simulink model "controller1"  (R2022a)
settings: Solver=VariableStepAuto  StartTime=0.0  StopTime=44  MaxStep=1e-3  MinStep=1e-6  RelTol=1e-3
libraries: dspswit3 x1
(part 2 of 2)

== matlab function controller1/Subsystem/MATLAB Function ==
  data: q input; f_matrix output; qd input; g_matrix output
function [f_matrix,g_matrix] = fcn(q,qd)
% q1=q(1);
q2=q(2);q3=q(3);
dq1=qd(1);dq2=qd(2);dq3=qd(3);

Izz1=0.192;
Ixx3=0.063; Iyy3=0.061; Izz3= 0.02;
Ixx2=0.0027; Iyy2=0.0024; Izz2=0.0004;

g_matrix =[                                                                                                                                                                                                                                                                                                                                                                                                                                                                                                                                                                                                                                                                                                                                                                                                                                                                                                                                                                                                                                                                                             0,                                                                                                                                                                                                             -(- sin(q2)*dq1^2*cos(q2)*sin(q3)^2 + sin(q2)*dq1^2*cos(q2) + dq2*cos(q3)*sin(q2)*dq1*cos(q2)^2*sin(q3) + dq2*sin(q2)*dq1*cos(q2)*sin(q3)^2 - dq2*sin(q2)*dq1*cos(q2))/(Iyy3*Izz1*Izz3 + Izz1*Izz2*Izz3 + Ixx2*Iyy3*Izz3*cos(q2)^2 + Ixx2*Izz2*Izz3*cos(q2)^2 + Ixx3*Izz1*Izz3*sin(q3)^2 + Iyy2*Iyy3*Izz3*sin(q2)^2 + Iyy2*Izz2*Izz3*sin(q2)^2 - Iyy3*Izz1*Izz3*sin(q3)^2 + Iyy3^2*Izz3*cos(q2)^2*sin(q3)^2 - Iyy3^2*Izz3*cos(q2)^2*sin(q3)^4 + Ixx3*Iyy3*Izz3*cos(q2)^2*cos(q3)^2 + Ixx3*Izz2*Izz3*cos(q2)^2*cos(q3)^2 + Ixx2*Ixx3*Izz3*cos(q2)^2*sin(q3)^2 - Ixx2*Iyy3*Izz3*cos(q2)^2*sin(q3)^2 + Ixx3*Iyy3*Izz3*cos(q2)^2*sin(q3)^4 + Iyy3*Izz2*Izz3*cos(q2)^2*sin(q3)^2 + Ixx3*Iyy2*Izz3*sin(q2)^2*sin(q3)^2 - Iyy2*Iyy3*Izz3*sin(q2)^2*sin(q3)^2 - Iyy3^2*Izz3*cos(q2)^2*cos(q3)^2*sin(q3)^2 + Ixx3*Iyy3*Izz3*cos(q2)^2*cos(q3)^2*sin(q3)^2),                                                                    (dq1^2*cos(q2)*sin(q2) - (dq1*dq2*cos(q2))/2 + (dq1*dq3*cos(q2))/2 - dq1^2*cos(q2)*sin(q2)*sin(q3)^2 + (dq1*dq2*cos(q2)*sin(q3)^2)/2 - (dq1*dq3*cos(q2)*sin(q3)^2)/2 - dq1*dq2*cos(q2)*sin(q2) - (dq1*dq3*cos(q2)*sin(q2))/2 + (dq2*dq3*cos(q2)*sin(q2))/2 + (dq1*dq2*cos(q2)^2*cos(q3)*sin(q3))/2 + (dq2*dq3*cos(q2)^2*cos(q3)*sin(q3))/2 + dq1*dq2*cos(q2)*sin(q2)*sin(q3)^2 + (dq1*dq3*cos(q2)*sin(q2)*sin(q3)^2)/2 - (dq2*dq3*cos(q2)*sin(q2)*sin(q3)^2)/2 + dq1*dq2*cos(q2)^2*cos(q3)*sin(q2)*sin(q3))/(Iyy3*Izz1*Izz3 + Izz1*Izz2*Izz3 + Ixx2*Iyy3*Izz3*cos(q2)^2 + Ixx2*Izz2*Izz3*cos(q2)^2 + Ixx3*Izz1*Izz3*sin(q3)^2 + Iyy2*Iyy3*Izz3*sin(q2)^2 + Iyy2*Izz2*Izz3*sin(q2)^2 - Iyy3*Izz1*Izz3*sin(q3)^2 + Iyy3^2*Izz3*cos(q2)^2*sin(q3)^2 - Iyy3^2*Izz3*cos(q2)^2*sin(q3)^4 + Ixx3*Iyy3*Izz3*cos(q2)^2*cos(q3)^2 + Ixx3*Izz2*Izz3*cos(q2)^2*cos(q3)^2 + Ixx2*Ixx3*Izz3*cos(q2)^2*sin(q3)^2 - Ixx2*Iyy3*Izz3*cos(q2)^2*sin(q3)^2 + Ixx3*Iyy3*Izz3*cos(q2)^2*sin(q3)^4 + Iyy3*Izz2*Izz3*cos(q2)^2*sin(q3)^2 + Ixx3*Iyy2*Izz3*sin(q2)^2*sin(q3)^2 - Iyy2*Iyy3*Izz3*sin(q2)^2*sin(q3)^2 - Iyy3^2*Izz3*cos(q2)^2*cos(q3)^2*sin(q3)^2 + Ixx3*Iyy3*Izz3*cos(q2)^2*cos(q3)^2*sin(q3)^2),                                                                                                                                                                                                                                                                                                                                                                                                                                                                                                                                                                                                                                                                                                                                                                                                                                            0,                                                                                                                                                                                                  (dq1*dq2*cos(q2)*sin(q2)*sin(q3)^2 - dq1^2*cos(q2)*sin(q2)*sin(q3)^2 + dq1*dq2*cos(q2)^2*cos(q3)*sin(q2)*sin(q3))/(Iyy3*Izz1*Izz3 + Izz1*Izz2*Izz3 + Ixx2*Iyy3*Izz3*cos(q2)^2 + Ixx2*Izz2*Izz3*cos(q2)^2 + Ixx3*Izz1*Izz3*sin(q3)^2 + Iyy2*Iyy3*Izz3*sin(q2)^2 + Iyy2*Izz2*Izz3*sin(q2)^2 - Iyy3*Izz1*Izz3*sin(q3)^2 + Iyy3^2*Izz3*cos(q2)^2*sin(q3)^2 - Iyy3^2*Izz3*cos(q2)^2*sin(q3)^4 + Ixx3*Iyy3*Izz3*cos(q2)^2*cos(q3)^2 + Ixx3*Izz2*Izz3*cos(q2)^2*cos(q3)^2 + Ixx2*Ixx3*Izz3*cos(q2)^2*sin(q3)^2 - Ixx2*Iyy3*Izz3*cos(q2)^2*sin(q3)^2 + Ixx3*Iyy3*Izz3*cos(q2)^2*sin(q3)^4 + Iyy3*Izz2*Izz3*cos(q2)^2*sin(q3)^2 + Ixx3*Iyy2*Izz3*sin(q2)^2*sin(q3)^2 - Iyy2*Iyy3*Izz3*sin(q2)^2*sin(q3)^2 - Iyy3^2*Izz3*cos(q2)^2*cos(q3)^2*sin(q3)^2 + Ixx3*Iyy3*Izz3*cos(q2)^2*cos(q3)^2*sin(q3)^2),                                                                                                                                                                                                                                                                                                       -(dq1*dq2*cos(q2)*sin(q2)*sin(q3)^2 - dq1^2*cos(q2)*sin(q2)*sin(q3)^2 + dq1*dq2*cos(q2)^2*cos(q3)*sin(q2)*sin(q3))/(Iyy3*Izz1*Izz3 + Izz1*Izz2*Izz3 + Ixx2*Iyy3*Izz3*cos(q2)^2 + Ixx2*Izz2*Izz3*cos(q2)^2 + Ixx3*Izz1*Izz3*sin(q3)^2 + Iyy2*Iyy3*Izz3*sin(q2)^2 + Iyy2*Izz2*Izz3*sin(q2)^2 - Iyy3*Izz1*Izz3*sin(q3)^2 + Iyy3^2*Izz3*cos(q2)^2*sin(q3)^2 - Iyy3^2*Izz3*cos(q2)^2*sin(q3)^4 + Ixx3*Iyy3*Izz3*cos(q2)^2*cos(q3)^2 + Ixx3*Izz2*Izz3*cos(q2)^2*cos(q3)^2 + Ixx2*Ixx3*Izz3*cos(q2)^2*sin(q3)^2 - Ixx2*Iyy3*Izz3*cos(q2)^2*sin(q3)^2 + Ixx3*Iyy3*Izz3*cos(q2)^2*sin(q3)^4 + Iyy3*Izz2*Izz3*cos(q2)^2*sin(q3)^2 + Ixx3*Iyy2*Izz3*sin(q2)^2*sin(q3)^2 - Iyy2*Iyy3*Izz3*sin(q2)^2*sin(q3)^2 - Iyy3^2*Izz3*cos(q2)^2*cos(q3)^2*sin(q3)^2 + Ixx3*Iyy3*Izz3*cos(q2)^2*cos(q3)^2*sin(q3)^2),                                                                      (cos(q2)*sin(q2)*dq1^2 - dq2*cos(q2)*sin(q2)*dq1)/(Iyy3*Izz1*Izz3 + Izz1*Izz2*Izz3 + Ixx2*Iyy3*Izz3*cos(q2)^2 + Ixx2*Izz2*Izz3*cos(q2)^2 + Ixx3*Izz1*Izz3*sin(q3)^2 + Iyy2*Iyy3*Izz3*sin(q2)^2 + Iyy2*Izz2*Izz3*sin(q2)^2 - Iyy3*Izz1*Izz3*sin(q3)^2 + Iyy3^2*Izz3*cos(q2)^2*sin(q3)^2 - Iyy3^2*Izz3*cos(q2)^2*sin(q3)^4 + Ixx3*Iyy3*Izz3*cos(q2)^2*cos(q3)^2 + Ixx3*Izz2*Izz3*cos(q2)^2*cos(q3)^2 + Ixx2*Ixx3*Izz3*cos(q2)^2*sin(q3)^2 - Ixx2*Iyy3*Izz3*cos(q2)^2*sin(q3)^2 + Ixx3*Iyy3*Izz3*cos(q2)^2*sin(q3)^4 + Iyy3*Izz2*Izz3*cos(q2)^2*sin(q3)^2 + Ixx3*Iyy2*Izz3*sin(q2)^2*sin(q3)^2 - Iyy2*Iyy3*Izz3*sin(q2)^2*sin(q3)^2 - Iyy3^2*Izz3*cos(q2)^2*cos(q3)^2*sin(q3)^2 + Ixx3*Iyy3*Izz3*cos(q2)^2*cos(q3)^2*sin(q3)^2)
                                                                                                                                                                                                                                                                                                                                                                                                                                                                                                                                                                                                                                                                                                                                                                                                                                                                                                                                                                                                                                                                                             0, -((dq2*dq3*cos(q2)^3)/2 - (dq1*dq2*cos(q2)^3)/2 + dq2^2*cos(q2)^2*cos(q3)*sin(q3) + dq1*dq2*cos(q2)^3*sin(q2) + dq1*dq2*cos(q2)^3*cos(q3)^2 - dq2*dq3*cos(q2)^3*cos(q3)^2 - dq2*dq3*cos(q2)^2*cos(q3)*sin(q3) - dq1*dq2*cos(q2)^3*cos(q3)^2*sin(q2) + dq1*dq2*cos(q2)^3*sin(q2)*sin(q3)^2 + dq1^2*cos(q2)^2*cos(q3)*sin(q2)*sin(q3) - 2*dq1*dq2*cos(q2)^2*cos(q3)*sin(q2)*sin(q3))/(Iyy3*Izz1*Izz3 + Izz1*Izz2*Izz3 + Ixx2*Iyy3*Izz3*cos(q2)^2 + Ixx2*Izz2*Izz3*cos(q2)^2 + Ixx3*Izz1*Izz3*sin(q3)^2 + Iyy2*Iyy3*Izz3*sin(q2)^2 + Iyy2*Izz2*Izz3*sin(q2)^2 - Iyy3*Izz1*Izz3*sin(q3)^2 + Iyy3^2*Izz3*cos(q2)^2*sin(q3)^2 - Iyy3^2*Izz3*cos(q2)^2*sin(q3)^4 + Ixx3*Iyy3*Izz3*cos(q2)^2*cos(q3)^2 + Ixx3*Izz2*Izz3*cos(q2)^2*cos(q3)^2 + Ixx2*Ixx3*Izz3*cos(q2)^2*sin(q3)^2 - Ixx2*Iyy3*Izz3*cos(q2)^2*sin(q3)^2 + Ixx3*Iyy3*Izz3*cos(q2)^2*sin(q3)^4 + Iyy3*Izz2*Izz3*cos(q2)^2*sin(q3)^2 + Ixx3*Iyy2*Izz3*sin(q2)^2*sin(q3)^2 - Iyy2*Iyy3*Izz3*sin(q2)^2*sin(q3)^2 - Iyy3^2*Izz3*cos(q2)^2*cos(q3)^2*sin(q3)^2 + Ixx3*Iyy3*Izz3*cos(q2)^2*cos(q3)^2*sin(q3)^2),                                                                                                                                                                                                ((dq1*dq2*cos(q2)^3*sin(q3)^2)/2 + (dq2*dq3*cos(q2)^3*sin(q3)^2)/2 - (dq1*dq2*cos(q2)^2*cos(q3)*sin(q3))/2 + (dq1*dq3*cos(q2)^2*cos(q3)*sin(q3))/2 + dq1*dq2*cos(q2)^3*sin(q2)*sin(q3)^2 + dq1^2*cos(q2)^2*cos(q3)*sin(q2)*sin(q3) - dq1*dq2*cos(q2)^2*cos(q3)*sin(q2)*sin(q3) - (dq1*dq3*cos(q2)^2*cos(q3)*sin(q2)*sin(q3))/2 + (dq2*dq3*cos(q2)^2*cos(q3)*sin(q2)*sin(q3))/2)/(Iyy3*Izz1*Izz3 + Izz1*Izz2*Izz3 + Ixx2*Iyy3*Izz3*cos(q2)^2 + Ixx2*Izz2*Izz3*cos(q2)^2 + Ixx3*Izz1*Izz3*sin(q3)^2 + Iyy2*Iyy3*Izz3*sin(q2)^2 + Iyy2*Izz2*Izz3*sin(q2)^2 - Iyy3*Izz1*Izz3*sin(q3)^2 + Iyy3^2*Izz3*cos(q2)^2*sin(q3)^2 - Iyy3^2*Izz3*cos(q2)^2*sin(q3)^4 + Ixx3*Iyy3*Izz3*cos(q2)^2*cos(q3)^2 + Ixx3*Izz2*Izz3*cos(q2)^2*cos(q3)^2 + Ixx2*Ixx3*Izz3*cos(q2)^2*sin(q3)^2 - Ixx2*Iyy3*Izz3*cos(q2)^2*sin(q3)^2 + Ixx3*Iyy3*Izz3*cos(q2)^2*sin(q3)^4 + Iyy3*Izz2*Izz3*cos(q2)^2*sin(q3)^2 + Ixx3*Iyy2*Izz3*sin(q2)^2*sin(q3)^2 - Iyy2*Iyy3*Izz3*sin(q2)^2*sin(q3)^2 - Iyy3^2*Izz3*cos(q2)^2*cos(q3)^2*sin(q3)^2 + Ixx3*Iyy3*Izz3*cos(q2)^2*cos(q3)^2*sin(q3)^2),                                                                                                                                                                                                                                                                                                                                                                                                                                                                                                                                                                                                                                                                                                                                                                                                                                            0, -((dq1*dq2*cos(q2)^3)/2 - (dq2*dq3*cos(q2)^3)/2 - dq2^2*cos(q2)^2*cos(q3)*sin(q3) - dq1*dq2*cos(q2)^3*cos(q3)^2 + dq2*dq3*cos(q2)^3*cos(q3)^2 + dq2*dq3*cos(q2)^2*cos(q3)*sin(q3) + 2*dq1*dq2*cos(q2)^3*cos(q3)^2*sin(q2) - dq1^2*cos(q2)^2*cos(q3)*sin(q2)*sin(q3) + 2*dq1*dq2*cos(q2)^2*cos(q3)*sin(q2)*sin(q3))/(Iyy3*Izz1*Izz3 + Izz1*Izz2*Izz3 + Ixx2*Iyy3*Izz3*cos(q2)^2 + Ixx2*Izz2*Izz3*cos(q2)^2 + Ixx3*Izz1*Izz3*sin(q3)^2 + Iyy2*Iyy3*Izz3*sin(q2)^2 + Iyy2*Izz2*Izz3*sin(q2)^2 - Iyy3*Izz1*Izz3*sin(q3)^2 + Iyy3^2*Izz3*cos(q2)^2*sin(q3)^2 - Iyy3^2*Izz3*cos(q2)^2*sin(q3)^4 + Ixx3*Iyy3*Izz3*cos(q2)^2*cos(q3)^2 + Ixx3*Izz2*Izz3*cos(q2)^2*cos(q3)^2 + Ixx2*Ixx3*Izz3*cos(q2)^2*sin(q3)^2 - Ixx2*Iyy3*Izz3*cos(q2)^2*sin(q3)^2 + Ixx3*Iyy3*Izz3*cos(q2)^2*sin(q3)^4 + Iyy3*Izz2*Izz3*cos(q2)^2*sin(q3)^2 + Ixx3*Iyy2*Izz3*sin(q2)^2*sin(q3)^2 - Iyy2*Iyy3*Izz3*sin(q2)^2*sin(q3)^2 - Iyy3^2*Izz3*cos(q2)^2*cos(q3)^2*sin(q3)^2 + Ixx3*Iyy3*Izz3*cos(q2)^2*cos(q3)^2*sin(q3)^2), -((dq1*dq2*cos(q2)*sin(q2)^2)/2 - dq2^2*cos(q3)*sin(q2)^2*sin(q3) - (dq2*dq3*cos(q2)*sin(q2)^2)/2 + dq1*dq2*cos(q3)*sin(q2)^3*sin(q3) + dq2*dq3*cos(q3)*sin(q2)^2*sin(q3) - dq1*dq2*cos(q2)*cos(q3)^2*sin(q2)^2 + dq1*dq2*cos(q2)*cos(q3)^2*sin(q2)^3 - dq1*dq2*cos(q2)^3*cos(q3)^2*sin(q2) + dq2*dq3*cos(q2)*cos(q3)^2*sin(q2)^2 + dq1^2*cos(q2)^2*cos(q3)*sin(q2)*sin(q3) - dq1*dq2*cos(q2)^2*cos(q3)*sin(q2)*sin(q3))/(Iyy3*Izz1*Izz3 + Izz1*Izz2*Izz3 + Ixx2*Iyy3*Izz3*cos(q2)^2 + Ixx2*Izz2*Izz3*cos(q2)^2 + Ixx3*Izz1*Izz3*sin(q3)^2 + Iyy2*Iyy3*Izz3*sin(q2)^2 + Iyy2*Izz2*Izz3*sin(q2)^2 - Iyy3*Izz1*Izz3*sin(q3)^2 + Iyy3^2*Izz3*cos(q2)^2*sin(q3)^2 - Iyy3^2*Izz3*cos(q2)^2*sin(q3)^4 + Ixx3*Iyy3*Izz3*cos(q2)^2*cos(q3)^2 + Ixx3*Izz2*Izz3*cos(q2)^2*cos(q3)^2 + Ixx2*Ixx3*Izz3*cos(q2)^2*sin(q3)^2 - Ixx2*Iyy3*Izz3*cos(q2)^2*sin(q3)^2 + Ixx3*Iyy3*Izz3*cos(q2)^2*sin(q3)^4 + Iyy3*Izz2*Izz3*cos(q2)^2*sin(q3)^2 + Ixx3*Iyy2*Izz3*sin(q2)^2*sin(q3)^2 - Iyy2*Iyy3*Izz3*sin(q2)^2*sin(q3)^2 - Iyy3^2*Izz3*cos(q2)^2*cos(q3)^2*sin(q3)^2 + Ixx3*Iyy3*Izz3*cos(q2)^2*cos(q3)^2*sin(q3)^2),                                                                                                                                                                                                                                                                                                                                                                                                                                                                                                                                                                                                                                                                                                                                                                                                 0
((dq1*dq3*cos(q2)^3)/2 + (dq2*dq3*cos(q2)^3)/2 - dq1*dq3*cos(q2)^3*cos(q3)^2 - dq2*dq3*cos(q2)^3*cos(q3)^2 - (dq1*dq3*cos(q2)^3*sin(q3)^2)/2 - (dq2*dq3*cos(q2)^3*sin(q3)^2)/2 - dq2*dq3*cos(q2)^2*cos(q3)*sin(q3) + dq1*dq3*cos(q2)^4*cos(q3)*sin(q3) + dq2*dq3*cos(q2)^2*cos(q3)*sin(q3)^3 - dq1*dq3*cos(q2)^4*cos(q3)*sin(q3)^3 + dq1*dq3*cos(q2)^3*cos(q3)^2*sin(q3)^2 + dq2*dq3*cos(q2)^3*cos(q3)^2*sin(q3)^2)/(Iyy3*Izz1*Izz3 + Izz1*Izz2*Izz3 + Ixx2*Iyy3*Izz3*cos(q2)^2 + Ixx2*Izz2*Izz3*cos(q2)^2 + Ixx3*Izz1*Izz3*sin(q3)^2 + Iyy2*Iyy3*Izz3*sin(q2)^2 + Iyy2*Izz2*Izz3*sin(q2)^2 - Iyy3*Izz1*Izz3*sin(q3)^2 + Iyy3^2*Izz3*cos(q2)^2*sin(q3)^2 - Iyy3^2*Izz3*cos(q2)^2*sin(q3)^4 + Ixx3*Iyy3*Izz3*cos(q2)^2*cos(q3)^2 + Ixx3*Izz2*Izz3*cos(q2)^2*cos(q3)^2 + Ixx2*Ixx3*Izz3*cos(q2)^2*sin(q3)^2 - Ixx2*Iyy3*Izz3*cos(q2)^2*sin(q3)^2 + Ixx3*Iyy3*Izz3*cos(q2)^2*sin(q3)^4 + Iyy3*Izz2*Izz3*cos(q2)^2*sin(q3)^2 + Ixx3*Iyy2*Izz3*sin(q2)^2*sin(q3)^2 - Iyy2*Iyy3*Izz3*sin(q2)^2*sin(q3)^2 - Iyy3^2*Izz3*cos(q2)^2*cos(q3)^2*sin(q3)^2 + Ixx3*Iyy3*Izz3*cos(q2)^2*cos(q3)^2*sin(q3)^2),                                                                                  (dq1^2*cos(q2)*sin(q2)^2 + (dq1*dq3*cos(q2)^3)/2 - (dq2*dq3*cos(q2)^3)/2 - dq1*dq2*cos(q2)*sin(q2)^2 - dq1^2*cos(q2)*sin(q2)^2*sin(q3)^2 - (dq1*dq3*cos(q2)^3*sin(q3)^2)/2 + (dq2*dq3*cos(q2)^3*sin(q3)^2)/2 + dq1*dq2*cos(q2)*sin(q2)^2*sin(q3)^2 + dq1*dq2*cos(q2)^2*cos(q3)*sin(q2)^2*sin(q3))/(Iyy3*Izz1*Izz3 + Izz1*Izz2*Izz3 + Ixx2*Iyy3*Izz3*cos(q2)^2 + Ixx2*Izz2*Izz3*cos(q2)^2 + Ixx3*Izz1*Izz3*sin(q3)^2 + Iyy2*Iyy3*Izz3*sin(q2)^2 + Iyy2*Izz2*Izz3*sin(q2)^2 - Iyy3*Izz1*Izz3*sin(q3)^2 + Iyy3^2*Izz3*cos(q2)^2*sin(q3)^2 - Iyy3^2*Izz3*cos(q2)^2*sin(q3)^4 + Ixx3*Iyy3*Izz3*cos(q2)^2*cos(q3)^2 + Ixx3*Izz2*Izz3*cos(q2)^2*cos(q3)^2 + Ixx2*Ixx3*Izz3*cos(q2)^2*sin(q3)^2 - Ixx2*Iyy3*Izz3*cos(q2)^2*sin(q3)^2 + Ixx3*Iyy3*Izz3*cos(q2)^2*sin(q3)^4 + Iyy3*Izz2*Izz3*cos(q2)^2*sin(q3)^2 + Ixx3*Iyy2*Izz3*sin(q2)^2*sin(q3)^2 - Iyy2*Iyy3*Izz3*sin(q2)^2*sin(q3)^2 - Iyy3^2*Izz3*cos(q2)^2*cos(q3)^2*sin(q3)^2 + Ixx3*Iyy3*Izz3*cos(q2)^2*cos(q3)^2*sin(q3)^2), -(dq1^2*cos(q2)*sin(q2)^2 - dq1*dq2*cos(q2)*sin(q2)^2 - (dq1*dq3*cos(q2)*sin(q2)^2)/2 + (dq2*dq3*cos(q2)*sin(q2)^2)/2 - dq1^2*cos(q2)*sin(q2)^2*sin(q3)^2 - (dq1*dq2*cos(q2)*sin(q2))/2 + (dq1*dq3*cos(q2)*sin(q2))/2 + (dq1*dq2*cos(q2)*sin(q2)*sin(q3)^2)/2 - (dq1*dq3*cos(q2)*sin(q2)*sin(q3)^2)/2 + dq1*dq2*cos(q2)*sin(q2)^2*sin(q3)^2 + (dq1*dq3*cos(q2)*sin(q2)^2*sin(q3)^2)/2 - (dq2*dq3*cos(q2)*sin(q2)^2*sin(q3)^2)/2 + dq1*dq2*cos(q2)^2*cos(q3)*sin(q2)^2*sin(q3) + (dq1*dq2*cos(q2)^2*cos(q3)*sin(q2)*sin(q3))/2 + (dq2*dq3*cos(q2)^2*cos(q3)*sin(q2)*sin(q3))/2)/(Iyy3*Izz1*Izz3 + Izz1*Izz2*Izz3 + Ixx2*Iyy3*Izz3*cos(q2)^2 + Ixx2*Izz2*Izz3*cos(q2)^2 + Ixx3*Izz1*Izz3*sin(q3)^2 + Iyy2*Iyy3*Izz3*sin(q2)^2 + Iyy2*Izz2*Izz3*sin(q2)^2 - Iyy3*Izz1*Izz3*sin(q3)^2 + Iyy3^2*Izz3*cos(q2)^2*sin(q3)^2 - Iyy3^2*Izz3*cos(q2)^2*sin(q3)^4 + Ixx3*Iyy3*Izz3*cos(q2)^2*cos(q3)^2 + Ixx3*Izz2*Izz3*cos(q2)^2*cos(q3)^2 + Ixx2*Ixx3*Izz3*cos(q2)^2*sin(q3)^2 - Ixx2*Iyy3*Izz3*cos(q2)^2*sin(q3)^2 + Ixx3*Iyy3*Izz3*cos(q2)^2*sin(q3)^4 + Iyy3*Izz2*Izz3*cos(q2)^2*sin(q3)^2 + Ixx3*Iyy2*Izz3*sin(q2)^2*sin(q3)^2 - Iyy2*Iyy3*Izz3*sin(q2)^2*sin(q3)^2 - Iyy3^2*Izz3*cos(q2)^2*cos(q3)^2*sin(q3)^2 + Ixx3*Iyy3*Izz3*cos(q2)^2*cos(q3)^2*sin(q3)^2), ((dq1*dq3*cos(q2))/2 + (dq2*dq3*cos(q2))/2 - dq1*dq3*cos(q2)*cos(q3)^2 - dq2*dq3*cos(q2)*cos(q3)^2 - dq2*dq3*cos(q3)*sin(q3) + dq1*dq3*cos(q2)^2*cos(q3)*sin(q3))/(Iyy3*Izz1*Izz3 + Izz1*Izz2*Izz3 + Ixx2*Iyy3*Izz3*cos(q2)^2 + Ixx2*Izz2*Izz3*cos(q2)^2 + Ixx3*Izz1*Izz3*sin(q3)^2 + Iyy2*Iyy3*Izz3*sin(q2)^2 + Iyy2*Izz2*Izz3*sin(q2)^2 - Iyy3*Izz1*Izz3*sin(q3)^2 + Iyy3^2*Izz3*cos(q2)^2*sin(q3)^2 - Iyy3^2*Izz3*cos(q2)^2*sin(q3)^4 + Ixx3*Iyy3*Izz3*cos(q2)^2*cos(q3)^2 + Ixx3*Izz2*Izz3*cos(q2)^2*cos(q3)^2 + Ixx2*Ixx3*Izz3*cos(q2)^2*sin(q3)^2 - Ixx2*Iyy3*Izz3*cos(q2)^2*sin(q3)^2 + Ixx3*Iyy3*Izz3*cos(q2)^2*sin(q3)^4 + Iyy3*Izz2*Izz3*cos(q2)^2*sin(q3)^2 + Ixx3*Iyy2*Izz3*sin(q2)^2*sin(q3)^2 - Iyy2*Iyy3*Izz3*sin(q2)^2*sin(q3)^2 - Iyy3^2*Izz3*cos(q2)^2*cos(q3)^2*sin(q3)^2 + Ixx3*Iyy3*Izz3*cos(q2)^2*cos(q3)^2*sin(q3)^2),                                                                                                                       -((dq2*dq3*cos(q2)^3*sin(q3)^2)/2 - (dq1*dq3*cos(q2)^3*sin(q3)^2)/2 - dq1^2*cos(q2)*sin(q2)^2*sin(q3)^2 + dq1*dq2*cos(q2)*sin(q2)^2*sin(q3)^2 + dq1*dq2*cos(q2)^2*cos(q3)*sin(q2)^2*sin(q3))/(Iyy3*Izz1*Izz3 + Izz1*Izz2*Izz3 + Ixx2*Iyy3*Izz3*cos(q2)^2 + Ixx2*Izz2*Izz3*cos(q2)^2 + Ixx3*Izz1*Izz3*sin(q3)^2 + Iyy2*Iyy3*Izz3*sin(q2)^2 + Iyy2*Izz2*Izz3*sin(q2)^2 - Iyy3*Izz1*Izz3*sin(q3)^2 + Iyy3^2*Izz3*cos(q2)^2*sin(q3)^2 - Iyy3^2*Izz3*cos(q2)^2*sin(q3)^4 + Ixx3*Iyy3*Izz3*cos(q2)^2*cos(q3)^2 + Ixx3*Izz2*Izz3*cos(q2)^2*cos(q3)^2 + Ixx2*Ixx3*Izz3*cos(q2)^2*sin(q3)^2 - Ixx2*Iyy3*Izz3*cos(q2)^2*sin(q3)^2 + Ixx3*Iyy3*Izz3*cos(q2)^2*sin(q3)^4 + Iyy3*Izz2*Izz3*cos(q2)^2*sin(q3)^2 + Ixx3*Iyy2*Izz3*sin(q2)^2*sin(q3)^2 - Iyy2*Iyy3*Izz3*sin(q2)^2*sin(q3)^2 - Iyy3^2*Izz3*cos(q2)^2*cos(q3)^2*sin(q3)^2 + Ixx3*Iyy3*Izz3*cos(q2)^2*cos(q3)^2*sin(q3)^2),                                                                                                                                                                                                              (dq1*dq2*cos(q2)*sin(q2)^2*sin(q3)^2 - dq1^2*cos(q2)*sin(q2)^2*sin(q3)^2 + (dq1*dq3*cos(q2)*sin(q2)^2*sin(q3)^2)/2 - (dq2*dq3*cos(q2)*sin(q2)^2*sin(q3)^2)/2 + dq1*dq2*cos(q2)^2*cos(q3)*sin(q2)^2*sin(q3))/(Iyy3*Izz1*Izz3 + Izz1*Izz2*Izz3 + Ixx2*Iyy3*Izz3*cos(q2)^2 + Ixx2*Izz2*Izz3*cos(q2)^2 + Ixx3*Izz1*Izz3*sin(q3)^2 + Iyy2*Iyy3*Izz3*sin(q2)^2 + Iyy2*Izz2*Izz3*sin(q2)^2 - Iyy3*Izz1*Izz3*sin(q3)^2 + Iyy3^2*Izz3*cos(q2)^2*sin(q3)^2 - Iyy3^2*Izz3*cos(q2)^2*sin(q3)^4 + Ixx3*Iyy3*Izz3*cos(q2)^2*cos(q3)^2 + Ixx3*Izz2*Izz3*cos(q2)^2*cos(q3)^2 + Ixx2*Ixx3*Izz3*cos(q2)^2*sin(q3)^2 - Ixx2*Iyy3*Izz3*cos(q2)^2*sin(q3)^2 + Ixx3*Iyy3*Izz3*cos(q2)^2*sin(q3)^4 + Iyy3*Izz2*Izz3*cos(q2)^2*sin(q3)^2 + Ixx3*Iyy2*Izz3*sin(q2)^2*sin(q3)^2 - Iyy2*Iyy3*Izz3*sin(q2)^2*sin(q3)^2 - Iyy3^2*Izz3*cos(q2)^2*cos(q3)^2*sin(q3)^2 + Ixx3*Iyy3*Izz3*cos(q2)^2*cos(q3)^2*sin(q3)^2), -(dq1^2*cos(q2)*sin(q2)^2 - dq1*dq2*cos(q2)*sin(q2)^2 - (dq1*dq3*cos(q2)*sin(q2)^2)/2 + (dq2*dq3*cos(q2)*sin(q2)^2)/2)/(Iyy3*Izz1*Izz3 + Izz1*Izz2*Izz3 + Ixx2*Iyy3*Izz3*cos(q2)^2 + Ixx2*Izz2*Izz3*cos(q2)^2 + Ixx3*Izz1*Izz3*sin(q3)^2 + Iyy2*Iyy3*Izz3*sin(q2)^2 + Iyy2*Izz2*Izz3*sin(q2)^2 - Iyy3*Izz1*Izz3*sin(q3)^2 + Iyy3^2*Izz3*cos(q2)^2*sin(q3)^2 - Iyy3^2*Izz3*cos(q2)^2*sin(q3)^4 + Ixx3*Iyy3*Izz3*cos(q2)^2*cos(q3)^2 + Ixx3*Izz2*Izz3*cos(q2)^2*cos(q3)^2 + Ixx2*Ixx3*Izz3*cos(q2)^2*sin(q3)^2 - Ixx2*Iyy3*Izz3*cos(q2)^2*sin(q3)^2 + Ixx3*Iyy3*Izz3*cos(q2)^2*sin(q3)^4 + Iyy3*Izz2*Izz3*cos(q2)^2*sin(q3)^2 + Ixx3*Iyy2*Izz3*sin(q2)^2*sin(q3)^2 - Iyy2*Iyy3*Izz3*sin(q2)^2*sin(q3)^2 - Iyy3^2*Izz3*cos(q2)^2*cos(q3)^2*sin(q3)^2 + Ixx3*Iyy3*Izz3*cos(q2)^2*cos(q3)^2*sin(q3)^2)];
 

f_matrix =[
                                                                                                                                                                                                                                                                                                                                                                                                                                                                                                                                                                                                                                                                                                                                                                                                                                                                                                                                                                                                                                                                                                                                                                                                                                                                                                                                                                                                                                                                                                                                                                                                                                                                                                                                                                                                                                                                                                                                                                                                                                                                                                                                                                                                                                                                                                                                                      -(dq1*((Izz3*dq1*(Iyy3 + Izz2 + Ixx3*sin(q3)^2 - Iyy3*sin(q3)^2)*(Ixx3*sin(2*q2 + 2*q3) - Iyy3*sin(2*q2 + 2*q3) + 2*Ixx2*sin(2*q2) + Ixx3*sin(2*q2) + Ixx3*sin(2*q3) - 2*Iyy2*sin(2*q2) + Iyy3*sin(2*q2) - Iyy3*sin(2*q3) - 2*Izz3*sin(2*q2)))/4 + (Izz3*dq3*cos(q2)*sin(q2)*(Iyy3 + Izz2 + Ixx3*sin(q3)^2 - Iyy3*sin(q3)^2)*(Iyy3 - Ixx3 + Izz3 + 2*Ixx3*cos(q3)^2 - 2*Iyy3*cos(q3)^2 - 2*Ixx3*cos(q2)*cos(q3)*sin(q3) + 2*Iyy3*cos(q2)*cos(q3)*sin(q3)))/2 + (Izz3*dq2*cos(q2)*cos(q3)*sin(q3)*(Ixx3 - Iyy3)*(2*Izz3*cos(q2) - 2*Ixx2*sin(2*q2) - Ixx3*sin(2*q2) + 2*Iyy2*sin(2*q2) - Iyy3*sin(2*q2) + 2*Izz3*sin(2*q2) - Ixx3*cos(2*q3)*sin(2*q2) + Iyy3*cos(2*q3)*sin(2*q2) + 2*Ixx3*cos(2*q3)*cos(q2) - 2*Iyy3*cos(2*q3)*cos(q2) - 2*Ixx3*sin(2*q3)*sin(q2) + 2*Iyy3*sin(2*q3)*sin(q2)))/4) + dq2*((Izz3*dq1*cos(q2)*(Iyy3 + Izz2 + Ixx3*sin(q3)^2 - Iyy3*sin(q3)^2)*(Ixx3 - Iyy3 + Izz3 - 2*Ixx2*sin(q2) + 2*Iyy2*sin(q2) - 2*Iyy3*sin(q2) + 2*Izz3*sin(q2) - 2*Ixx3*cos(q3)^2 + 2*Iyy3*cos(q3)^2 - 2*Ixx3*cos(q3)^2*sin(q2) + 2*Iyy3*cos(q3)^2*sin(q2)))/2 - (Izz3*dq3*sin(q2)*(Iyy3 + Izz2 + Ixx3*sin(q3)^2 - Iyy3*sin(q3)^2)*(Ixx3*cos(q2) - Iyy3*cos(q2) + Izz3*cos(q2) - Ixx3*sin(2*q3) + Iyy3*sin(2*q3) - 2*Ixx3*cos(q2)*cos(q3)^2 + 2*Iyy3*cos(q2)*cos(q3)^2))/2 + (Izz3*dq2*sin(2*q3)*cos(q2)*cos(q3)*sin(q3)*(Ixx3 - Iyy3)^2)/2) - dq3*((Izz3*dq1*cos(q2)*(Iyy3 + Izz2 + Ixx3*sin(q3)^2 - Iyy3*sin(q3)^2)*(Ixx3 - Iyy3 + Izz3 - 2*Ixx3*cos(q3)^2 + 2*Iyy3*cos(q3)^2 + 2*Ixx3*cos(q2)*cos(q3)*sin(q3) - 2*Iyy3*cos(q2)*cos(q3)*sin(q3)))/2 - (Izz3*dq2*cos(q2)*cos(q3)*sin(q3)*(Ixx3 - Iyy3)*(Ixx3*cos(q2) - Iyy3*cos(q2) + Izz3*cos(q2) - Ixx3*sin(2*q3) + Iyy3*sin(2*q3) - 2*Ixx3*cos(q2)*cos(q3)^2 + 2*Iyy3*cos(q2)*cos(q3)^2))/2) + Iyy3*Izz3^2*(dq1^2*cos(q2)*sin(q2) - (dq1*dq2*cos(q2))/2 + (dq1*dq3*cos(q2))/2 - dq1^2*cos(q2)*sin(q2)*sin(q3)^2 + (dq1*dq2*cos(q2)*sin(q3)^2)/2 - (dq1*dq3*cos(q2)*sin(q3)^2)/2 - dq1*dq2*cos(q2)*sin(q2) - (dq1*dq3*cos(q2)*sin(q2))/2 + (dq2*dq3*cos(q2)*sin(q2))/2 + (dq1*dq2*cos(q2)^2*cos(q3)*sin(q3))/2 + (dq2*dq3*cos(q2)^2*cos(q3)*sin(q3))/2 + dq1*dq2*cos(q2)*sin(q2)*sin(q3)^2 + (dq1*dq3*cos(q2)*sin(q2)*sin(q3)^2)/2 - (dq2*dq3*cos(q2)*sin(q2)*sin(q3)^2)/2 + dq1*dq2*cos(q2)^2*cos(q3)*sin(q2)*sin(q3)) + Iyy2*Izz2*Izz3*(cos(q2)*sin(q2)*dq1^2 - dq2*cos(q2)*sin(q2)*dq1) - Ixx2*Iyy3*Izz3*(- sin(q2)*dq1^2*cos(q2)*sin(q3)^2 + sin(q2)*dq1^2*cos(q2) + dq2*cos(q3)*sin(q2)*dq1*cos(q2)^2*sin(q3) + dq2*sin(q2)*dq1*cos(q2)*sin(q3)^2 - dq2*sin(q2)*dq1*cos(q2)) + Ixx2*Ixx3*Izz3*(dq1*dq2*cos(q2)*sin(q2)*sin(q3)^2 - dq1^2*cos(q2)*sin(q2)*sin(q3)^2 + dq1*dq2*cos(q2)^2*cos(q3)*sin(q2)*sin(q3)) - Ixx3*Iyy2*Izz3*(dq1*dq2*cos(q2)*sin(q2)*sin(q3)^2 - dq1^2*cos(q2)*sin(q2)*sin(q3)^2 + dq1*dq2*cos(q2)^2*cos(q3)*sin(q2)*sin(q3)))/(Iyy3*Izz1*Izz3 + Izz1*Izz2*Izz3 + Ixx2*Iyy3*Izz3*cos(q2)^2 + Ixx2*Izz2*Izz3*cos(q2)^2 + Ixx3*Izz1*Izz3*sin(q3)^2 + Iyy2*Iyy3*Izz3*sin(q2)^2 + Iyy2*Izz2*Izz3*sin(q2)^2 - Iyy3*Izz1*Izz3*sin(q3)^2 + Iyy3^2*Izz3*cos(q2)^2*sin(q3)^2 - Iyy3^2*Izz3*cos(q2)^2*sin(q3)^4 + Ixx3*Iyy3*Izz3*cos(q2)^2*cos(q3)^2 + Ixx3*Izz2*Izz3*cos(q2)^2*cos(q3)^2 + Ixx2*Ixx3*Izz3*cos(q2)^2*sin(q3)^2 - Ixx2*Iyy3*Izz3*cos(q2)^2*sin(q3)^2 + Ixx3*Iyy3*Izz3*cos(q2)^2*sin(q3)^4 + Iyy3*Izz2*Izz3*cos(q2)^2*sin(q3)^2 + Ixx3*Iyy2*Izz3*sin(q2)^2*sin(q3)^2 - Iyy2*Iyy3*Izz3*sin(q2)^2*sin(q3)^2 - Iyy3^2*Izz3*cos(q2)^2*cos(q3)^2*sin(q3)^2 + Ixx3*Iyy3*Izz3*cos(q2)^2*cos(q3)^2*sin(q3)^2)
                                                                                                                                                                                                                                                                                                                                                                                                                                                                                                                                                                                                                                                                                                                                                                                                                                                                                                                                                                                                                                                                                                                                                                                                                                                                                                                                                                                                                                                                                                                                                                                                                                                     (dq1*((dq2*(Ixx3*Izz3*cos(q2)^2*cos(q3)^2 + Iyy3*Izz3*cos(q2)^2*sin(q3)^2 + Ixx2*Izz3*cos(q2)^2 + Iyy2*Izz3*sin(q2)^2 + Izz1*Izz3)*(2*Izz3*cos(q2) - 2*Ixx2*sin(2*q2) - Ixx3*sin(2*q2) + 2*Iyy2*sin(2*q2) - Iyy3*sin(2*q2) + 2*Izz3*sin(2*q2) - Ixx3*cos(2*q3)*sin(2*q2) + Iyy3*cos(2*q3)*sin(2*q2) + 2*Ixx3*cos(2*q3)*cos(q2) - 2*Iyy3*cos(2*q3)*cos(q2) - 2*Ixx3*sin(2*q3)*sin(q2) + 2*Iyy3*sin(2*q3)*sin(q2)))/4 + (Izz3*dq1*cos(q2)*cos(q3)*sin(q3)*(Ixx3 - Iyy3)*(Ixx3*sin(2*q2 + 2*q3) - Iyy3*sin(2*q2 + 2*q3) + 2*Ixx2*sin(2*q2) + Ixx3*sin(2*q2) + Ixx3*sin(2*q3) - 2*Iyy2*sin(2*q2) + Iyy3*sin(2*q2) - Iyy3*sin(2*q3) - 2*Izz3*sin(2*q2)))/4 + (Izz3*dq3*cos(q2)^2*cos(q3)*sin(q2)*sin(q3)*(Ixx3 - Iyy3)*(Iyy3 - Ixx3 + Izz3 + 2*Ixx3*cos(q3)^2 - 2*Iyy3*cos(q3)^2 - 2*Ixx3*cos(q2)*cos(q3)*sin(q3) + 2*Iyy3*cos(q2)*cos(q3)*sin(q3)))/2) + dq2*((dq2*sin(2*q3)*(Ixx3 - Iyy3)*(Ixx3*Izz3*cos(q2)^2*cos(q3)^2 + Iyy3*Izz3*cos(q2)^2*sin(q3)^2 + Ixx2*Izz3*cos(q2)^2 + Iyy2*Izz3*sin(q2)^2 + Izz1*Izz3))/2 + (Izz3*dq1*cos(q2)^2*cos(q3)*sin(q3)*(Ixx3 - Iyy3)*(Ixx3 - Iyy3 + Izz3 - 2*Ixx2*sin(q2) + 2*Iyy2*sin(q2) - 2*Iyy3*sin(q2) + 2*Izz3*sin(q2) - 2*Ixx3*cos(q3)^2 + 2*Iyy3*cos(q3)^2 - 2*Ixx3*cos(q3)^2*sin(q2) + 2*Iyy3*cos(q3)^2*sin(q2)))/2 - (Izz3*dq3*cos(q2)*cos(q3)*sin(q2)*sin(q3)*(Ixx3 - Iyy3)*(Ixx3*cos(q2) - Iyy3*cos(q2) + Izz3*cos(q2) - Ixx3*sin(2*q3) + Iyy3*sin(2*q3) - 2*Ixx3*cos(q2)*cos(q3)^2 + 2*Iyy3*cos(q2)*cos(q3)^2))/2) + dq3*((dq2*(Ixx3*Izz3*cos(q2)^2*cos(q3)^2 + Iyy3*Izz3*cos(q2)^2*sin(q3)^2 + Ixx2*Izz3*cos(q2)^2 + Iyy2*Izz3*sin(q2)^2 + Izz1*Izz3)*(Ixx3*cos(q2) - Iyy3*cos(q2) + Izz3*cos(q2) - Ixx3*sin(2*q3) + Iyy3*sin(2*q3) - 2*Ixx3*cos(q2)*cos(q3)^2 + 2*Iyy3*cos(q2)*cos(q3)^2))/2 - (Izz3*dq1*cos(q2)^2*cos(q3)*sin(q3)*(Ixx3 - Iyy3)*(Ixx3 - Iyy3 + Izz3 - 2*Ixx3*cos(q3)^2 + 2*Iyy3*cos(q3)^2 + 2*Ixx3*cos(q2)*cos(q3)*sin(q3) - 2*Iyy3*cos(q2)*cos(q3)*sin(q3)))/2) - Iyy3*Izz3^2*((dq1*dq2*cos(q2)^3*sin(q3)^2)/2 + (dq2*dq3*cos(q2)^3*sin(q3)^2)/2 - (dq1*dq2*cos(q2)^2*cos(q3)*sin(q3))/2 + (dq1*dq3*cos(q2)^2*cos(q3)*sin(q3))/2 + dq1*dq2*cos(q2)^3*sin(q2)*sin(q3)^2 + dq1^2*cos(q2)^2*cos(q3)*sin(q2)*sin(q3) - dq1*dq2*cos(q2)^2*cos(q3)*sin(q2)*sin(q3) - (dq1*dq3*cos(q2)^2*cos(q3)*sin(q2)*sin(q3))/2 + (dq2*dq3*cos(q2)^2*cos(q3)*sin(q2)*sin(q3))/2) + Ixx3*Iyy2*Izz3*((dq1*dq2*cos(q2)*sin(q2)^2)/2 - dq2^2*cos(q3)*sin(q2)^2*sin(q3) - (dq2*dq3*cos(q2)*sin(q2)^2)/2 + dq1*dq2*cos(q3)*sin(q2)^3*sin(q3) + dq2*dq3*cos(q3)*sin(q2)^2*sin(q3) - dq1*dq2*cos(q2)*cos(q3)^2*sin(q2)^2 + dq1*dq2*cos(q2)*cos(q3)^2*sin(q2)^3 - dq1*dq2*cos(q2)^3*cos(q3)^2*sin(q2) + dq2*dq3*cos(q2)*cos(q3)^2*sin(q2)^2 + dq1^2*cos(q2)^2*cos(q3)*sin(q2)*sin(q3) - dq1*dq2*cos(q2)^2*cos(q3)*sin(q2)*sin(q3)) + Ixx2*Iyy3*Izz3*((dq2*dq3*cos(q2)^3)/2 - (dq1*dq2*cos(q2)^3)/2 + dq2^2*cos(q2)^2*cos(q3)*sin(q3) + dq1*dq2*cos(q2)^3*sin(q2) + dq1*dq2*cos(q2)^3*cos(q3)^2 - dq2*dq3*cos(q2)^3*cos(q3)^2 - dq2*dq3*cos(q2)^2*cos(q3)*sin(q3) - dq1*dq2*cos(q2)^3*cos(q3)^2*sin(q2) + dq1*dq2*cos(q2)^3*sin(q2)*sin(q3)^2 + dq1^2*cos(q2)^2*cos(q3)*sin(q2)*sin(q3) - 2*dq1*dq2*cos(q2)^2*cos(q3)*sin(q2)*sin(q3)) + Ixx2*Ixx3*Izz3*((dq1*dq2*cos(q2)^3)/2 - (dq2*dq3*cos(q2)^3)/2 - dq2^2*cos(q2)^2*cos(q3)*sin(q3) - dq1*dq2*cos(q2)^3*cos(q3)^2 + dq2*dq3*cos(q2)^3*cos(q3)^2 + dq2*dq3*cos(q2)^2*cos(q3)*sin(q3) + 2*dq1*dq2*cos(q2)^3*cos(q3)^2*sin(q2) - dq1^2*cos(q2)^2*cos(q3)*sin(q2)*sin(q3) + 2*dq1*dq2*cos(q2)^2*cos(q3)*sin(q2)*sin(q3)))/(Iyy3*Izz1*Izz3 + Izz1*Izz2*Izz3 + Ixx2*Iyy3*Izz3*cos(q2)^2 + Ixx2*Izz2*Izz3*cos(q2)^2 + Ixx3*Izz1*Izz3*sin(q3)^2 + Iyy2*Iyy3*Izz3*sin(q2)^2 + Iyy2*Izz2*Izz3*sin(q2)^2 - Iyy3*Izz1*Izz3*sin(q3)^2 + Iyy3^2*Izz3*cos(q2)^2*sin(q3)^2 - Iyy3^2*Izz3*cos(q2)^2*sin(q3)^4 + Ixx3*Iyy3*Izz3*cos(q2)^2*cos(q3)^2 + Ixx3*Izz2*Izz3*cos(q2)^2*cos(q3)^2 + Ixx2*Ixx3*Izz3*cos(q2)^2*sin(q3)^2 - Ixx2*Iyy3*Izz3*cos(q2)^2*sin(q3)^2 + Ixx3*Iyy3*Izz3*cos(q2)^2*sin(q3)^4 + Iyy3*Izz2*Izz3*cos(q2)^2*sin(q3)^2 + Ixx3*Iyy2*Izz3*sin(q2)^2*sin(q3)^2 - Iyy2*Iyy3*Izz3*sin(q2)^2*sin(q3)^2 - Iyy3^2*Izz3*cos(q2)^2*cos(q3)^2*sin(q3)^2 + Ixx3*Iyy3*Izz3*cos(q2)^2*cos(q3)^2*sin(q3)^2)
(dq1*((dq3*cos(q2)*(Iyy3 - Ixx3 + Izz3 + 2*Ixx3*cos(q3)^2 - 2*Iyy3*cos(q3)^2 - 2*Ixx3*cos(q2)*cos(q3)*sin(q3) + 2*Iyy3*cos(q2)*cos(q3)*sin(q3))*(Iyy3*Izz1 + Izz1*Izz2 + Ixx2*Iyy3*cos(q2)^2 + Ixx2*Izz2*cos(q2)^2 + Ixx3*Izz1*sin(q3)^2 + Iyy2*Iyy3*sin(q2)^2 + Iyy2*Izz2*sin(q2)^2 - Iyy3*Izz1*sin(q3)^2 + Iyy3*Izz3*sin(q2)^2 + Izz2*Izz3*sin(q2)^2 + Iyy3^2*cos(q2)^2*sin(q3)^2 - Iyy3^2*cos(q2)^2*sin(q3)^4 + Ixx3*Iyy3*cos(q2)^2*cos(q3)^2 + Ixx3*Izz2*cos(q2)^2*cos(q3)^2 + Ixx2*Ixx3*cos(q2)^2*sin(q3)^2 - Ixx2*Iyy3*cos(q2)^2*sin(q3)^2 + Ixx3*Iyy3*cos(q2)^2*sin(q3)^4 + Iyy3*Izz2*cos(q2)^2*sin(q3)^2 + Ixx3*Iyy2*sin(q2)^2*sin(q3)^2 - Iyy2*Iyy3*sin(q2)^2*sin(q3)^2 + Ixx3*Izz3*sin(q2)^2*sin(q3)^2 - Iyy3*Izz3*sin(q2)^2*sin(q3)^2 - Iyy3^2*cos(q2)^2*cos(q3)^2*sin(q3)^2 + Ixx3*Iyy3*cos(q2)^2*cos(q3)^2*sin(q3)^2))/2 + (Izz3*dq1*sin(q2)*(Iyy3 + Izz2 + Ixx3*sin(q3)^2 - Iyy3*sin(q3)^2)*(Ixx3*sin(2*q2 + 2*q3) - Iyy3*sin(2*q2 + 2*q3) + 2*Ixx2*sin(2*q2) + Ixx3*sin(2*q2) + Ixx3*sin(2*q3) - 2*Iyy2*sin(2*q2) + Iyy3*sin(2*q2) - Iyy3*sin(2*q3) - 2*Izz3*sin(2*q2)))/4 + (Izz3*dq2*cos(q2)*cos(q3)*sin(q2)*sin(q3)*(Ixx3 - Iyy3)*(2*Izz3*cos(q2) - 2*Ixx2*sin(2*q2) - Ixx3*sin(2*q2) + 2*Iyy2*sin(2*q2) - Iyy3*sin(2*q2) + 2*Izz3*sin(2*q2) - Ixx3*cos(2*q3)*sin(2*q2) + Iyy3*cos(2*q3)*sin(2*q2) + 2*Ixx3*cos(2*q3)*cos(q2) - 2*Iyy3*cos(2*q3)*cos(q2) - 2*Ixx3*sin(2*q3)*sin(q2) + 2*Iyy3*sin(2*q3)*sin(q2)))/4) - dq3*((Izz3*dq1*cos(q2)*sin(q2)*(Iyy3 + Izz2 + Ixx3*sin(q3)^2 - Iyy3*sin(q3)^2)*(Ixx3 - Iyy3 + Izz3 - 2*Ixx3*cos(q3)^2 + 2*Iyy3*cos(q3)^2 + 2*Ixx3*cos(q2)*cos(q3)*sin(q3) - 2*Iyy3*cos(q2)*cos(q3)*sin(q3)))/2 - (Izz3*dq2*cos(q2)*cos(q3)*sin(q2)*sin(q3)*(Ixx3 - Iyy3)*(Ixx3*cos(q2) - Iyy3*cos(q2) + Izz3*cos(q2) - Ixx3*sin(2*q3) + Iyy3*sin(2*q3) - 2*Ixx3*cos(q2)*cos(q3)^2 + 2*Iyy3*cos(q2)*cos(q3)^2))/2) + dq2*((Izz3*dq1*cos(q2)*sin(q2)*(Iyy3 + Izz2 + Ixx3*sin(q3)^2 - Iyy3*sin(q3)^2)*(Ixx3 - Iyy3 + Izz3 - 2*Ixx2*sin(q2) + 2*Iyy2*sin(q2) - 2*Iyy3*sin(q2) + 2*Izz3*sin(q2) - 2*Ixx3*cos(q3)^2 + 2*Iyy3*cos(q3)^2 - 2*Ixx3*cos(q3)^2*sin(q2) + 2*Iyy3*cos(q3)^2*sin(q2)))/2 - (dq3*(Ixx3*cos(q2) - Iyy3*cos(q2) + Izz3*cos(q2) - Ixx3*sin(2*q3) + Iyy3*sin(2*q3) - 2*Ixx3*cos(q2)*cos(q3)^2 + 2*Iyy3*cos(q2)*cos(q3)^2)*(Iyy3*Izz1 + Izz1*Izz2 + Ixx2*Iyy3*cos(q2)^2 + Ixx2*Izz2*cos(q2)^2 + Ixx3*Izz1*sin(q3)^2 + Iyy2*Iyy3*sin(q2)^2 + Iyy2*Izz2*sin(q2)^2 - Iyy3*Izz1*sin(q3)^2 + Iyy3*Izz3*sin(q2)^2 + Izz2*Izz3*sin(q2)^2 + Iyy3^2*cos(q2)^2*sin(q3)^2 - Iyy3^2*cos(q2)^2*sin(q3)^4 + Ixx3*Iyy3*cos(q2)^2*cos(q3)^2 + Ixx3*Izz2*cos(q2)^2*cos(q3)^2 + Ixx2*Ixx3*cos(q2)^2*sin(q3)^2 - Ixx2*Iyy3*cos(q2)^2*sin(q3)^2 + Ixx3*Iyy3*cos(q2)^2*sin(q3)^4 + Iyy3*Izz2*cos(q2)^2*sin(q3)^2 + Ixx3*Iyy2*sin(q2)^2*sin(q3)^2 - Iyy2*Iyy3*sin(q2)^2*sin(q3)^2 + Ixx3*Izz3*sin(q2)^2*sin(q3)^2 - Iyy3*Izz3*sin(q2)^2*sin(q3)^2 - Iyy3^2*cos(q2)^2*cos(q3)^2*sin(q3)^2 + Ixx3*Iyy3*cos(q2)^2*cos(q3)^2*sin(q3)^2))/2 + (Izz3*dq2*sin(2*q3)*cos(q2)*cos(q3)*sin(q2)*sin(q3)*(Ixx3 - Iyy3)^2)/2) + Iyy3*Izz3^2*(dq1^2*cos(q2)*sin(q2)^2 - dq1*dq2*cos(q2)*sin(q2)^2 - (dq1*dq3*cos(q2)*sin(q2)^2)/2 + (dq2*dq3*cos(q2)*sin(q2)^2)/2 - dq1^2*cos(q2)*sin(q2)^2*sin(q3)^2 - (dq1*dq2*cos(q2)*sin(q2))/2 + (dq1*dq3*cos(q2)*sin(q2))/2 + (dq1*dq2*cos(q2)*sin(q2)*sin(q3)^2)/2 - (dq1*dq3*cos(q2)*sin(q2)*sin(q3)^2)/2 + dq1*dq2*cos(q2)*sin(q2)^2*sin(q3)^2 + (dq1*dq3*cos(q2)*sin(q2)^2*sin(q3)^2)/2 - (dq2*dq3*cos(q2)*sin(q2)^2*sin(q3)^2)/2 + dq1*dq2*cos(q2)^2*cos(q3)*sin(q2)^2*sin(q3) + (dq1*dq2*cos(q2)^2*cos(q3)*sin(q2)*sin(q3))/2 + (dq2*dq3*cos(q2)^2*cos(q3)*sin(q2)*sin(q3))/2) - Ixx2*Iyy3^2*((dq1*dq3*cos(q2)^3)/2 + (dq2*dq3*cos(q2)^3)/2 - dq1*dq3*cos(q2)^3*cos(q3)^2 - dq2*dq3*cos(q2)^3*cos(q3)^2 - (dq1*dq3*cos(q2)^3*sin(q3)^2)/2 - (dq2*dq3*cos(q2)^3*sin(q3)^2)/2 - dq2*dq3*cos(q2)^2*cos(q3)*sin(q3) + dq1*dq3*cos(q2)^4*cos(q3)*sin(q3) + dq2*dq3*cos(q2)^2*cos(q3)*sin(q3)^3 - dq1*dq3*cos(q2)^4*cos(q3)*sin(q3)^3 + dq1*dq3*cos(q2)^3*cos(q3)^2*sin(q3)^2 + dq2*dq3*cos(q2)^3*cos(q3)^2*sin(q3)^2) - Ixx3*Iyy2*Izz3*(dq1*dq2*cos(q2)*sin(q2)^2*sin(q3)^2 - dq1^2*cos(q2)*sin(q2)^2*sin(q3)^2 + (dq1*dq3*cos(q2)*sin(q2)^2*sin(q3)^2)/2 - (dq2*dq3*cos(q2)*sin(q2)^2*sin(q3)^2)/2 + dq1*dq2*cos(q2)^2*cos(q3)*sin(q2)^2*sin(q3)) + Ixx2*Ixx3*Izz3*((dq2*dq3*cos(q2)^3*sin(q3)^2)/2 - (dq1*dq3*cos(q2)^3*sin(q3)^2)/2 - dq1^2*cos(q2)*sin(q2)^2*sin(q3)^2 + dq1*dq2*cos(q2)*sin(q2)^2*sin(q3)^2 + dq1*dq2*cos(q2)^2*cos(q3)*sin(q2)^2*sin(q3)) - Ixx2*Iyy3*Izz3*(dq1^2*cos(q2)*sin(q2)^2 + (dq1*dq3*cos(q2)^3)/2 - (dq2*dq3*cos(q2)^3)/2 - dq1*dq2*cos(q2)*sin(q2)^2 - dq1^2*cos(q2)*sin(q2)^2*sin(q3)^2 - (dq1*dq3*cos(q2)^3*sin(q3)^2)/2 + (dq2*dq3*cos(q2)^3*sin(q3)^2)/2 + dq1*dq2*cos(q2)*sin(q2)^2*sin(q3)^2 + dq1*dq2*cos(q2)^2*cos(q3)*sin(q2)^2*sin(q3)) + Iyy2*Izz2*Izz3*(dq1^2*cos(q2)*sin(q2)^2 - dq1*dq2*cos(q2)*sin(q2)^2 - (dq1*dq3*cos(q2)*sin(q2)^2)/2 + (dq2*dq3*cos(q2)*sin(q2)^2)/2) - Iyy3*Izz1*Izz2*((dq1*dq3*cos(q2))/2 + (dq2*dq3*cos(q2))/2 - dq1*dq3*cos(q2)*cos(q3)^2 - dq2*dq3*cos(q2)*cos(q3)^2 - dq2*dq3*cos(q3)*sin(q3) + dq1*dq3*cos(q2)^2*cos(q3)*sin(q3)))/(Iyy3*Izz1*Izz3 + Izz1*Izz2*Izz3 + Ixx2*Iyy3*Izz3*cos(q2)^2 + Ixx2*Izz2*Izz3*cos(q2)^2 + Ixx3*Izz1*Izz3*sin(q3)^2 + Iyy2*Iyy3*Izz3*sin(q2)^2 + Iyy2*Izz2*Izz3*sin(q2)^2 - Iyy3*Izz1*Izz3*sin(q3)^2 + Iyy3^2*Izz3*cos(q2)^2*sin(q3)^2 - Iyy3^2*Izz3*cos(q2)^2*sin(q3)^4 + Ixx3*Iyy3*Izz3*cos(q2)^2*cos(q3)^2 + Ixx3*Izz2*Izz3*cos(q2)^2*cos(q3)^2 + Ixx2*Ixx3*Izz3*cos(q2)^2*sin(q3)^2 - Ixx2*Iyy3*Izz3*cos(q2)^2*sin(q3)^2 + Ixx3*Iyy3*Izz3*cos(q2)^2*sin(q3)^4 + Iyy3*Izz2*Izz3*cos(q2)^2*sin(q3)^2 + Ixx3*Iyy2*Izz3*sin(q2)^2*sin(q3)^2 - Iyy2*Iyy3*Izz3*sin(q2)^2*sin(q3)^2 - Iyy3^2*Izz3*cos(q2)^2*cos(q3)^2*sin(q3)^2 + Ixx3*Iyy3*Izz3*cos(q2)^2*cos(q3)^2*sin(q3)^2)];

== matlab function controller1/Subsystem/MATLAB Function1 ==
  data: p input; q input; Z output; G output
function [Z,G] = fcn(p,q)


Z=q'*p;
G=q'*q;

== matlab function controller1/Subsystem/MATLAB Function2 ==
  data: Z input; G input; teta_hat output; t input; dteta output
function [teta_hat,dteta] = fcn(Z,G,t)
T=4;
t_ti=0.81;
Izz1=0.192;
Ixx3=0.063; Iyy3=0.061; Izz3= 0.02;
Ixx2=0.0027; Iyy2=0.0024; Izz2=0.0004;
teta=[Ixx2*Iyy3^2
     Ixx2*Iyy3*Izz3
     Iyy3*Izz3^2
     Iyy3*Izz1*Izz2
     Ixx2*Ixx3*Izz3
     Ixx3*Iyy2*Izz3
     Iyy2*Izz2*Izz3];
Izz1=0.12;
Ixx3=0.051; Iyy3=0.1; Izz3= 0.2;
Ixx2=0.02; Iyy2=0.2; Izz2=0.001;




if t>t_ti
Izz1=0.162;
Ixx3=0.063; Iyy3=0.05; Izz3= 0.02;
Ixx2=0.0027; Iyy2=0.024; Izz2=0.0006;
end

if t>t_ti+T
Izz1=0.2;
Ixx3=0.063; Iyy3=0.055; Izz3= 0.02;
Ixx2=0.002; Iyy2=0.002; Izz2=0.0005;
end

if t>t_ti+2*T
Izz1=0.192;
Ixx3=0.063; Iyy3=0.061; Izz3= 0.02;
Ixx2=0.0027; Iyy2=0.0024; Izz2=0.0004;
end
teta_hat=[Ixx2*Iyy3^2
     Ixx2*Iyy3*Izz3
     Iyy3*Izz3^2
     Iyy3*Izz1*Izz2
     Ixx2*Ixx3*Izz3
     Ixx3*Iyy2*Izz3
     Iyy2*Izz2*Izz3];
dteta=teta_hat-teta;
% v=G\Z;
% minn=(v-teta_hat).^2;
% if ti==1 && t>0.3
% teta_hat=v;
% end

== matlab function controller1/Subsystem/MATLAB Function3 ==
  data: q input; Ve output; qd input; q_des input; qd_des input; q0_des input; qd0_des input; q0 input; qd0 input; timeofupdate input; ae output; ti output; t input
function [Ve,ae,ti] = fcn(q,qd,q_des,qd_des,q0_des,qd0_des,q0,qd0,timeofupdate,t)
ti=0;

e1=q-q_des;
e2=qd-qd_des;
e10=q0-q0_des;
e20=qd0-qd0_des;
v0=0.5*(e10(1)^2+e10(2)^2+e10(3)^2)+1.5*(e20(1)^2+e20(2)^2+e20(3)^2);
t0=0;
% if t==2
% v0=0.5*(e1(1)^2+e1(2)^2+e1(3)^2)+2.5*(e2(1)^2+e2(2)^2+e2(3)^2);
% t0=t;
% end

Ve=0.5*(e1(1)^2+e1(2)^2+e1(3)^2)+1.5*(e2(1)^2+e2(2)^2+e2(3)^2);
ae=0.5*(e1(1)^2+e1(2)^2+e1(3)^2)^2+(e2(1)^2+e2(2)^2+e2(3)^2)+v0;
% if timeofupdate>0
% t0=t;
% v0=Ve;
% end
if Ve>v0+ae || t>=t0+5
ti=1;%action
end
